simulink model "Final_JSB_4wp_LQG_withNoise_GnSch_Autopilotsbsy"  (R2025a)
settings: Solver=FixedStepDiscrete  StartTime=0.0  StopTime=600  FixedStep=0.008333  RelTol=1e-3
libraries: aerolibfltsims x1
settings Model: Creator=HP  LastModifiedBy=HP
settings DataIOCC: StreamToWks=off  ReturnWorkspaceOutputs=off

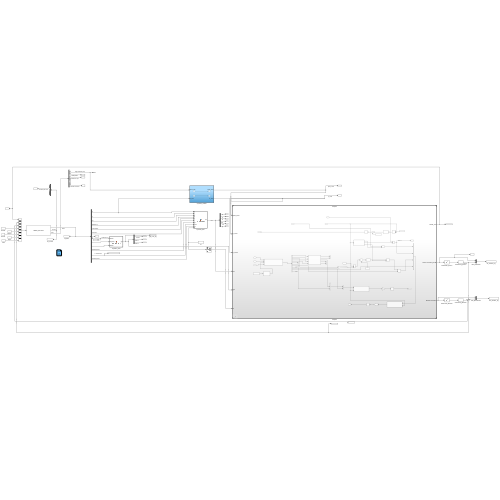
[thumbnail: Simulink's stored preview of the top-level diagram]
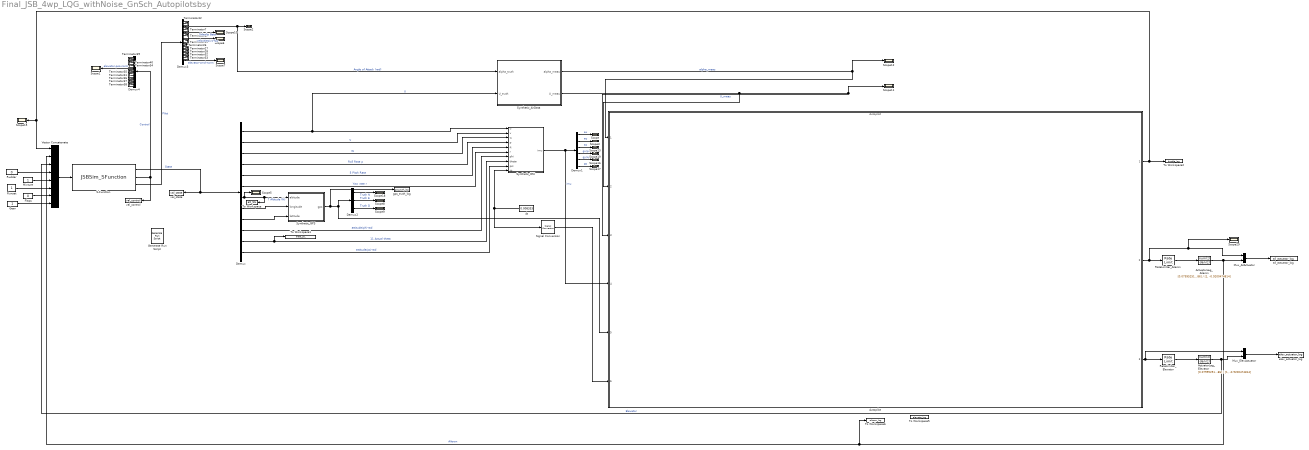
== system Final_JSB_4wp_LQG_withNoise_GnSch_Autopilotsbsy ==
  ActuatorLag_Aileron : DiscreteTransferFcn  Numerator=[0.0799525186]  Denominator=[1, -0.9200474814]
  ActuatorLag_Elevator : DiscreteTransferFcn  Numerator=[0.0799525186]  Denominator=[1, -0.9200474814]
  Autopilot : ModelReference  ModelNameDialog=Autopilot  SimulationMode=Normal  ModelReferenceVersion=1.490
  Demux : Demux  Outputs=12
  Demux1 : Demux  Outputs=6
  Demux2 : Demux  Outputs=3
  Demux3 : Demux  Outputs=13
  Demux4 : Demux  Outputs=9
  Flaps : Constant  Value=0  SampleTime=0.008333
  Gear : Constant  SampleTime=0.008333
  Generate Run Script : aerolibfltsims/Generate Run Script  Architecture=Win64  dataFlow=Send  GeometryModelName=c172p  AirportId=KSFO  RunwayId=10L  InitialAltitude=13  InitialHeading=113  OffsetDistance=4.72  OffsetAzimuth=0  InstallScenery=on  DisableShaders=off  OriginAddress=127.0.0.1  DestinationPort=5502  OriginPort=5505  LocalAddress=127.0.0.1  OutputFileName=runfg.bat  FlightGearBaseDirectory=D:\FlightGear 2024.1
  Mixture : Constant  SampleTime=0.008333
  Mux_AilActuator : Mux  Inputs=2
  Mux_ElevActuator : Mux  Inputs=2
  RateLimiter_Aileron : RateLimiter  SampleTimeMode=inherited
  RateLimiter_Elevator : RateLimiter  SampleTimeMode=inherited
  Rudder : Constant  Value=0  SampleTime=0.008333
  Runset : Constant  SampleTime=0.008333
  S-Function : S-Function  FunctionName=JSBSim_SFunction  Parameters='c172p',0.008333,1,'scripts/c172_cruise_8K_FINAL_FG','c172p_low_init','c172_simulink'  SFunctionDeploymentMode=off  EnableBusSupport=off
  Scope{,1..3,5..13,15..19,29} (19 alike) : Scope
      Scope settings: ActiveDisplayYMinimum=-1  ActiveDisplayYMaximum=1  DataLoggingVariableName=ScopeData10
      Scope1 settings: ActiveDisplayYMinimum=-1.1506994257290051  ActiveDisplayYMaximum=0.35818130652817959
      Scope10 settings: ActiveDisplayYMinimum=-0.013709260264701928  ActiveDisplayYMaximum=0.01519858722297282  DataLoggingVariableName=ScopeData7
      Scope11 settings: ActiveDisplayYMinimum=3415.5653951242566  ActiveDisplayYMaximum=9259.4920568838716  DataLoggingVariableName=ScopeData8
      Scope12 settings: ActiveDisplayYMinimum=3415.5653951242566  ActiveDisplayYMaximum=9259.4920568838716  DataLoggingVariableName=ScopeData9
      Scope13 settings: ActiveDisplayYMinimum=-1  ActiveDisplayYMaximum=1  DataLoggingVariableName=ScopeData12
      Scope15 settings: ActiveDisplayYMinimum=-0.018881594286629666  ActiveDisplayYMaximum=0.11615642817640902  DataLoggingVariableName=ScopeData26
      Scope16 settings: ActiveDisplayYMinimum=-1  ActiveDisplayYMaximum=1  DataLoggingVariableName=ScopeData14
      Scope17 settings: ActiveDisplayYMinimum=-1  ActiveDisplayYMaximum=1  DataLoggingVariableName=ScopeData15
      Scope18 settings: ActiveDisplayYMinimum=-26491.073215571287  ActiveDisplayYMaximum=2943.4525795079203  DataLoggingVariableName=ScopeData16
      Scope19 settings: ActiveDisplayYMinimum=-1  ActiveDisplayYMaximum=1  DataLoggingVariableName=ScopeData17
      Scope2 settings: ActiveDisplayYMinimum=-0.011798630048731329  ActiveDisplayYMaximum=0.11950334473381488
      Scope29 settings: ActiveDisplayYMinimum=-0.17748082414582364  ActiveDisplayYMaximum=0.3098920504311331  DataLoggingVariableName=ScopeData28
      Scope3 settings: ActiveDisplayYMinimum=-1  ActiveDisplayYMaximum=1  DataLoggingVariableName=ScopeData11
      Scope5 settings: ActiveDisplayYMinimum=3997.0534475268796  ActiveDisplayYMaximum=4001.1947988374159  DataLoggingVariableName=ScopeData32
      Scope6 settings: ActiveDisplayYMinimum=164.40851412581961  ActiveDisplayYMaximum=177.60462429694334  DataLoggingVariableName=ScopeData3
      Scope7 settings: ActiveDisplayYMinimum=-0.073115917661029928  ActiveDisplayYMaximum=0.2264682659900942  DataLoggingVariableName=ScopeData2
      Scope8 settings: ActiveDisplayYMinimum=-26491.073215571287  ActiveDisplayYMaximum=2943.4525795079203  DataLoggingVariableName=ScopeData5
      Scope9 settings: ActiveDisplayYMinimum=-26491.073215571287  ActiveDisplayYMaximum=2943.4525795079203  DataLoggingVariableName=ScopeData6
  Signal Conversion : SignalConversion  OverrideOpt=on
  Synthetic_AirData : Subsystem  TreatAsAtomicUnit=on
  Synthetic_GPS : MATLAB Function  TreatAsAtomicUnit=on  SystemSampleTime=0.008333
  Synthetic_IMU : MATLAB Function  TreatAsAtomicUnit=on  SystemSampleTime=0.008333
  Terminator{7,20,25..28,32..42} (17 alike) : Terminator
  To Workspace : ToWorkspace  VariableName=alt_SIL  SaveFormat=Timeseries  SampleTime=0.008333
  To Workspace1 : ToWorkspace  VariableName=theta_SIL  SaveFormat=Timeseries  SampleTime=0.008333
  To Workspace2 : ToWorkspace  VariableName=throttle_log  SaveFormat=Structure With Time  SampleTime=0.008333
  To Workspace5 : ToWorkspace  VariableName=elevator_log  SaveFormat=Structure With Time  SampleTime=0.008333
  To Workspace6 : ToWorkspace  VariableName=aileron_log  SaveFormat=Structure With Time  SampleTime=0.008333
  Vector Concatenate : Concatenate  NumInputs=8
  ail_actuator_log : ToWorkspace  VariableName=ail_actuator_log  SaveFormat=Structure With Time  SampleTime=0.008333
  dt : Constant  Value=0.008333  SampleTime=0.008333
  elev_actuator_log : ToWorkspace  VariableName=elev_actuator_log  SaveFormat=Structure With Time  SampleTime=0.008333
  gps_truth_log : ToWorkspace  VariableName=gps_truth_log  SaveFormat=Structure With Time  SampleTime=0.008333
  val_control : ToWorkspace  VariableName=val_control  SaveFormat=Structure With Time  SampleTime=0.008333
  val_state : ToWorkspace  VariableName=val_state  SaveFormat=Structure With Time  SampleTime=0.008333
  wires:
  Flaps/1 -> Vector Concatenate/7
  Runset/1 -> Vector Concatenate/6
  Vector Concatenate/1 -> S-Function/1
  Demux3/2 -> Scope2/1, Synthetic_AirData/1(alpha_truth)  "Angle of Attack (rad)"
  Mixture/1 -> Vector Concatenate/5
  Gear/1 -> Vector Concatenate/8
  Rudder/1 -> Vector Concatenate/4
  Demux/3 -> Synthetic_IMU/3(w)  "W"
  Demux/12 -> Synthetic_IMU/9(psi)  "attitude/psi-rad"
  Demux/2 -> Synthetic_IMU/2(v)  "V"
  Demux/4 -> Synthetic_IMU/4(p)  "Roll Rate p"
  Demux/6 -> Synthetic_IMU/6(r)  "Yaw rate r"
  Demux4/3 -> Terminator34/1
  S-Function/1 -> Demux/1, val_state/1  "State"
  Demux3/6 -> Scope6/1  "velocities/vc-fps"
  Demux3/7 -> Terminator25/1
  Demux4/9 -> Terminator38/1
  Demux3/3 -> Terminator7/1
  Demux3/10 -> Terminator28/1
  Demux4/5 -> Terminator35/1
  Demux3/11 -> Terminator32/1
  Demux3/4 -> Scope10/1  "Sideslip Beta"
  Demux4/4 -> Scope1/1  "elevator-pos-norm"
  Demux4/7 -> Terminator36/1
  Demux4/6 -> Terminator41/1
  Demux4/1 -> Terminator39/1
  Demux3/1 -> Terminator42/1
  Demux4/2 -> Terminator40/1
  Demux3/5 -> Terminator20/1
  Demux4/8 -> Terminator37/1
  Demux3/12 -> Terminator33/1
  Demux3/9 -> Terminator27/1
  Demux3/8 -> Terminator26/1
  S-Function/3 -> Demux3/1  "Pilot"
  Demux3/13 -> Scope7/1  "elevator-cmd-norm"
  S-Function/2 -> val_control/1, Demux4/1  "Control"
  Demux/1 -> Synthetic_AirData/2(U_truth), Synthetic_IMU/1(u)  "U"
  Demux/5 -> Synthetic_IMU/5(q)  "5 Pitch Rate"
  Demux/7 -> Scope5/1, To Workspace/1, Synthetic_GPS/1(altitude)  "7 Altitude (ft)"
  Demux/10 -> Synthetic_IMU/7(phi)  "attitude/phi-rad"
  Demux/11 -> To Workspace1/1, Synthetic_IMU/8(theta)  "11 Actual theta"
  Synthetic_IMU/1(imu) -> Autopilot/4, Demux1/1  "imu"
  Demux1/1 -> Scope/1  "ax"
  Demux1/2 -> Scope3/1  "ay"
  Demux1/3 -> Scope13/1  "az"
  Demux1/5 -> Scope16/1  "gy/q"
  Demux1/6 -> Scope17/1  "gz"
  Demux/8 -> Synthetic_GPS/2(longitude)
  Demux/9 -> Synthetic_GPS/3(latitude)
  Synthetic_GPS/1(gps) -> gps_truth_log/1, Autopilot/5, Demux2/1
  Demux2/1 -> Scope18/1  "Truth N"
  Demux2/2 -> Scope8/1  "Truth E"
  Demux2/3 -> Scope9/1  "Truth D"
  Synthetic_AirData/2(U_meas) -> Autopilot/2, Autopilot/3, Scope11/1  "U_meas"
  dt/1 -> Signal Conversion/1, Synthetic_IMU/10(dt)
  Synthetic_AirData/1(alpha_meas) -> Autopilot/1, Scope12/1  "alpha_meas"
  Demux1/4 -> Scope19/1  "gx/p"
  RateLimiter_Elevator/1 -> ActuatorLag_Elevator/1
  ActuatorLag_Elevator/1 -> Vector Concatenate/3, Mux_ElevActuator/2  "Elevator"
  RateLimiter_Aileron/1 -> ActuatorLag_Aileron/1
  ActuatorLag_Aileron/1 -> To Workspace6/1, Vector Concatenate/2, Mux_AilActuator/2  "Aileron"
  Mux_ElevActuator/1 -> elev_actuator_log/1
  Mux_AilActuator/1 -> ail_actuator_log/1
  Autopilot/3 -> RateLimiter_Elevator/1, Mux_ElevActuator/1
  Autopilot/1 -> Vector Concatenate/1, Scope15/1, To Workspace2/1
  Autopilot/2 -> RateLimiter_Aileron/1, Mux_AilActuator/1, Scope29/1
  Signal Conversion/1 -> Autopilot/6

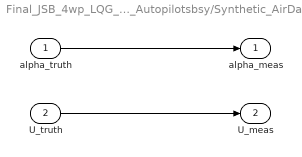
== system Final_JSB_4wp_LQG_withNoise_GnSch_Autopilotsbsy/Synthetic_AirData ==
  alpha_truth : Inport
  U_truth : Inport  Port=2
  alpha_meas : Outport
  U_meas : Outport  Port=2
  wires:
  U_truth/1 -> U_meas/1
  alpha_truth/1 -> alpha_meas/1

== matlab function Final_JSB_4wp_LQG_withNoise_GnSch_Autopilotsbsy/Synthetic_GPS ==
  data: altitude input; longitude input; latitude input; gps output
function gps = Synthetic_GPS(altitude,longitude , latitude)
%#codegen
%
% Synthetic GPS interface for JSBSim C172
%
% Inputs:
%   latitude  [deg]
%   longitude [deg]
%   altitude  [ft]
%
% Output:
%   gps = [north; east; down] [m]

% ---------------------------------------------------------
% Earth radius
% ---------------------------------------------------------
Re = 6371000.0;

% ---------------------------------------------------------
% Store initial GPS position
% ---------------------------------------------------------
persistent lat0 lon0 alt0 initialized

if isempty(initialized)

    lat0 = latitude;
    lon0 = longitude;
    alt0 = altitude;

    initialized = true;
end

% ---------------------------------------------------------
% Convert degrees to radians
% ---------------------------------------------------------
lat = latitude * pi / 180.0;
lon = longitude * pi / 180.0;

lat0_rad = lat0 * pi / 180.0;
lon0_rad = lon0 * pi / 180.0;

% ---------------------------------------------------------
% Local North position
% ---------------------------------------------------------
north = (lat - lat0_rad) * Re;

% ---------------------------------------------------------
% Local East position
% ---------------------------------------------------------
east = (lon - lon0_rad) * Re * cos(lat0_rad);

% ---------------------------------------------------------
% Down position
%
% JSBSim altitude is positive upward.
% NED Down is positive downward.
% ---------------------------------------------------------
down = -(altitude - alt0) * 0.3048;

% ---------------------------------------------------------
% GPS measurement
% ---------------------------------------------------------
gps = [north; east; down];

end

== matlab function Final_JSB_4wp_LQG_withNoise_GnSch_Autopilotsbsy/Synthetic_IMU ==
  data: u input; imu output; v input; w input; p input; q input; r input; phi input; theta input; psi input; dt input
function imu = Synthetic_IMU(u, v, w, p, q, r, ...
                             phi, theta, psi, dt)
%#codegen
%
% C172 Synthetic IMU
%
% Output:
%   imu = [ax ay az gx gy gz]
%
% Units:
%   acceleration : m/s^2
%   angular rate : rad/s
%
% Sensor model:
%   truth + zero-mean Gaussian measurement noise
%
% IMPORTANT:
%   This is a measurement model, not the aircraft dynamics model.

ENABLE_ACCEL_NOISE = true;
ENABLE_GYRO_NOISE  = true;

GRAVITY = 9.80665;

% =========================================================
% SENSOR NOISE PARAMETERS
% =========================================================
%
% These are INITIAL ENGINEERING DESIGN VALUES.
% They are NOT claimed to have been measured from the C172.
%
% They will be validated using the sensor-vs-truth residuals.
%

ACCEL_NOISE_STD = 0.03;      % m/s^2
GYRO_NOISE_STD  = 0.002;     % rad/s -- matches EKF R exactly, do not change
                              % one without updating the other.

% Optional constant biases.
% Start at zero so we isolate random measurement noise first.

ACCEL_BIAS = [0.0; 0.0; 0.0];    % m/s^2
GYRO_BIAS  = [0.0; 0.0; 0.0];    % rad/s


% =========================================================
% Convert JSBSim body velocity: ft/s -> m/s
% =========================================================

u = u * 0.3048;
v = v * 0.3048;
w = w * 0.3048;


% =========================================================
% Previous velocity
% =========================================================

persistent u_prev v_prev w_prev initialized

if isempty(initialized)

    u_prev = u;
    v_prev = v;
    w_prev = w;

    initialized = true;

end


% =========================================================
% Body translational velocity derivatives
% =========================================================

udot = (u - u_prev) / dt;
vdot = (v - v_prev) / dt;
wdot = (w - w_prev) / dt;


% =========================================================
% Body translational acceleration
% =========================================================

ax_body = udot + q*w - r*v;
ay_body = vdot + r*u - p*w;
az_body = wdot + p*v - q*u;

accel_body = [
    ax_body;
    ay_body;
    az_body
];


% =========================================================
% Body -> NED rotation
% =========================================================

cp = cos(phi);
sp = sin(phi);

ct = cos(theta);
st = sin(theta);

cy = cos(psi);
sy = sin(psi);

C_bn = [

    ct*cy, ...
    sp*st*cy - cp*sy, ...
    cp*st*cy + sp*sy;

    ct*sy, ...
    sp*st*sy + cp*cy, ...
    cp*st*sy - sp*cy;

    -st, ...
    sp*ct, ...
    cp*ct
];


% =========================================================
% Gravity
% =========================================================

gravity_ned = [
    0;
    0;
    GRAVITY
];

gravity_body = C_bn' * gravity_ned;


% =========================================================
% Specific force
% =========================================================

specific_force_body = ...
    accel_body - gravity_body;


% =========================================================
% TRUE IMU VALUES
% =========================================================

accel_true = specific_force_body;

gyro_true = [
    p;
    q;
    r
];


% =========================================================
% SENSOR MEASUREMENT NOISE
% =========================================================

if ENABLE_ACCEL_NOISE
    accel_noise = ACCEL_NOISE_STD * randn(3,1);
else
    accel_noise = zeros(3,1);
end

if ENABLE_GYRO_NOISE
    gyro_noise = GYRO_NOISE_STD * randn(3,1);
else
    gyro_noise = zeros(3,1);
end


% =========================================================
% SENSOR MEASUREMENTS
% =========================================================

accel_meas = ...
    accel_true + ACCEL_BIAS + accel_noise;

gyro_meas = ...
    gyro_true + GYRO_BIAS + gyro_noise;


% =========================================================
% Update previous velocity
% =========================================================

u_prev = u;
v_prev = v;
w_prev = w;


% =========================================================
% Output
% =========================================================

imu = [
    accel_meas(1);
    accel_meas(2);
    accel_meas(3);
    gyro_meas(1);
    gyro_meas(2);
    gyro_meas(3)
];

end
